simulink model "flyback_sim"  (R2021b)
settings: Solver=VariableStepAuto  StartTime=0  StopTime=0.1  FixedStep=0.00001  RelTol=1e-3
libraries: spsRMSLib x2, spsSeriesRLCBranchLib x2, spsCurrentMeasurementLib x1, spsDCVoltageSourceLib x1, spsDiodeLib x1, spsLinearTransformerLib x1, spsMosfetLib x1, spsVoltageMeasurementLib x1, spspowerguiLib x1
settings Model: Creator=Casper  LastModifiedBy=Casper

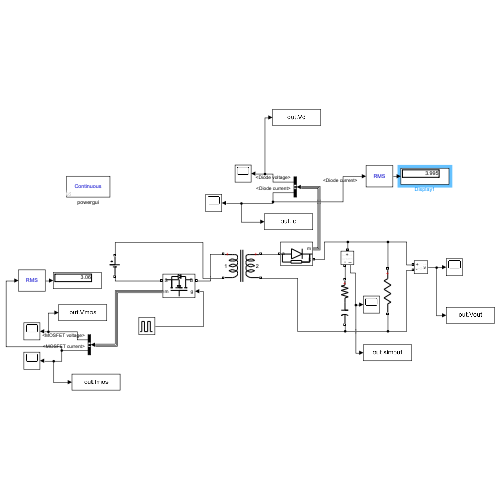
[thumbnail: Simulink's stored preview of the top-level diagram]
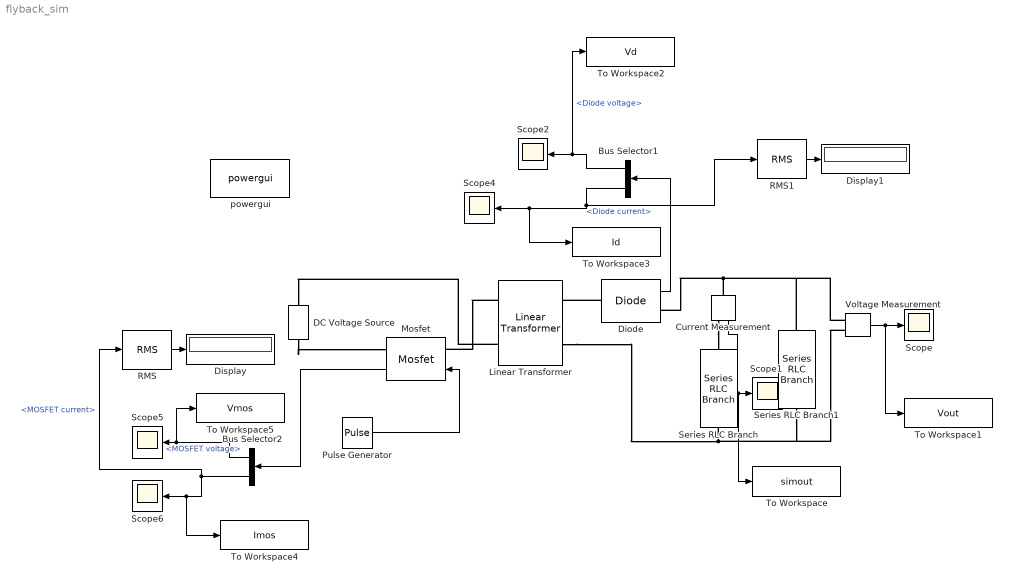
== system flyback_sim ==
  Bus Selector1 : BusSelector  OutputSignals=Diode voltage,Diode current
  Bus Selector2 : BusSelector  OutputSignals=MOSFET voltage,MOSFET current
  Current Measurement : spsCurrentMeasurementLib/Current Measurement  PhasorSimulation=off  OutputType=Complex  PSBequivalent=0
  DC Voltage Source : spsDCVoltageSourceLib/DC Voltage Source  Amplitude=24  Measurements=None
  Diode : spsDiodeLib/Diode  Ron=0.001  Lon=0  Vf=0.6  IC=0  UseSnubber=0  Rs=500  Cs=250e-9  Measurements=on
  Display : Display
  Display1 : Display
  Linear Transformer : spsLinearTransformerLib/Linear Transformer  UNITS=SI  NominalPower=[ 45 100e3 ]  winding1=[48 0 0]  winding2=[41.1428 0 0]  ThreeWindings=off  winding3=[3.15e+05 4.41e+06 280.75]  RmLm=[6400 0.01378]  Measurements=None  DataType=on
  Mosfet : spsMosfetLib/Mosfet  Ron=0.1  Lon=0  Rd=0.01  Vfd=0  IC=0  Rs=1e5  Cs=inf  Measurements=on
  Pulse Generator : DiscretePulseGenerator  PulseType=Time based  Period=1.25e-5  PulseWidth=43.75
  RMS : spsRMSLib/RMS  TrueRMS=on  Freq=60  RMSInit=120  Ts=0
  RMS1 : spsRMSLib/RMS  TrueRMS=on  Freq=60  RMSInit=120  Ts=0
  Scope{,1..2,4..6} (6 alike) : Scope
  Series RLC Branch : spsSeriesRLCBranchLib/Series RLC Branch  LConnTagsString=__new0  RConnTagsString=__new0  BranchType=RC  Resistance=0.05  Inductance=1e-3  SetiL0=off  InitialCurrent=0  Capacitance=100e-6  Setx0=off  InitialVoltage=0  Measurements=None
  Series RLC Branch1 : spsSeriesRLCBranchLib/Series RLC Branch  LConnTagsString=__new0  RConnTagsString=__new0  BranchType=R  Resistance=5  Inductance=1e-3  SetiL0=off  InitialCurrent=0  Capacitance=1e-6  Setx0=off  InitialVoltage=0  Measurements=None
  To Workspace : ToWorkspace  VariableName=simout  SaveFormat=Timeseries  SampleTime=-1
  To Workspace1 : ToWorkspace  VariableName=Vout  SaveFormat=Timeseries  SampleTime=-1
  To Workspace2 : ToWorkspace  VariableName=Vd  SaveFormat=Timeseries  SampleTime=-1
  To Workspace3 : ToWorkspace  VariableName=Id  SaveFormat=Timeseries  SampleTime=-1
  To Workspace4 : ToWorkspace  VariableName=Imos  SaveFormat=Timeseries  SampleTime=-1
  To Workspace5 : ToWorkspace  VariableName=Vmos  SaveFormat=Timeseries  SampleTime=-1
  Voltage Measurement : spsVoltageMeasurementLib/Voltage Measurement  PhasorSimulation=off  OutputType=Complex  PSBequivalent=0
  powergui : spspowerguiLib/powergui  Priority=1  SimulationMode=Continuous  SampleTime=1e-6  frequency=60  Iterations=50  frequencyindice=0  Pbase=100e6  ErrMax=1e-4  UnitsV=kV  UnitsW=MW  buscounter=0  FunctionMessages=off  echomessages=off  EnableUseOfTLC=off  CurrentSourceSwitches=off  DisableSnubberDevices=off  DisableRonSwitches=off  DisableVfSwitches=off  DisplayEquations=off  AutomaticDiscreteSolvers=off  SolverType=Tustin/Backward Euler (TBE)  Interpol=off  ExternalGateDelay=off  methode=off  Ts=100  x0status=blocks  SPID=on  SwTol=0  HookPort=off  NonlinearTolerance=1e-4  nMaxIteration=100  ContinueOnMaxIteration=off  RestoreLinks=warning  ResistiveCurrentMeasurement=off  Frange=[0:2:500]  Ylog=off  Xlog=on  ShowGrid=off  save=off  variable=ZData  structure=0  ZoomFFT=off  StartTime=0.0  cycles=1  DisplayStyle=1  fundamental=60  FreqAxis=off  MaxFrequency=1000  frequencyindicesteady=1  RmsSteady=1  display=off
  wires:
  Pulse Generator/1 -> Mosfet/1
  Voltage Measurement/1 -> To Workspace1/1, Scope/1
  Diode/1 -> Bus Selector1/1
  Bus Selector1/1 -> To Workspace2/1, Scope2/1  "<Diode voltage>"
  Bus Selector2/1 -> To Workspace5/1, Scope5/1  "<MOSFET voltage>"
  Bus Selector2/2 -> To Workspace4/1, Scope6/1, RMS/1  "<MOSFET current>"
  Mosfet/1 -> Bus Selector2/1
  RMS/1 -> Display/1
  Bus Selector1/2 -> RMS1/1, To Workspace3/1, Scope4/1  "<Diode current>"
  RMS1/1 -> Display1/1
  Current Measurement/1 -> To Workspace/1, Scope1/1
  connections:
  Diode/LConn1 -- Linear Transformer/RConn1
  Voltage Measurement/LConn1 -- Series RLC Branch1/LConn1 -- Current Measurement/LConn1 -- Diode/RConn1
  Linear Transformer/RConn2 -- Series RLC Branch/RConn1 -- Series RLC Branch1/RConn1 -- Voltage Measurement/LConn2
  DC Voltage Source/LConn1 -- Mosfet/RConn1
  Linear Transformer/LConn1 -- Mosfet/LConn1
  Linear Transformer/LConn2 -- DC Voltage Source/RConn1
  Current Measurement/RConn1 -- Series RLC Branch/LConn1
